simulink model "massignment2"  (Simulink 6.0)
settings: Solver=FixedStepDiscrete  StartTime=0.0  StopTime=10.0  RelTol=1e-3
settings Model: Creator=awarlock  LastModifiedBy=awarlock  ExtModeAutoUpdateStatusClock=off
settings OptimizationCC: InlineParams=on
settings DebuggingCC: MultiTaskDSMMsg=warning

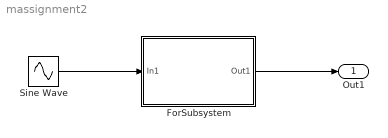
== system massignment2 ==
  ForSubsystem : Subsystem
  Sine Wave : Sin  Amplitude=3:7  SampleTime=0.1
  Out1 : Outport
  wires:
  Sine Wave/1 -> ForSubsystem/1(In1)
  ForSubsystem/1(Out1) -> Out1/1

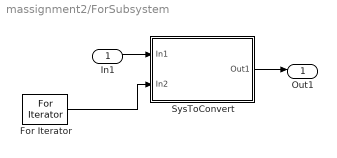
== system massignment2/ForSubsystem ==
  In1 : Inport  Port=1  LatchInput=off
  For Iterator : ForIterator  IterationVariableDataType=double
  SysToConvert : Subsystem  TreatAsAtomicUnit=on
  Out1 : Outport
  wires:
  In1/1 -> SysToConvert/1(In1)
  SysToConvert/1(Out1) -> Out1/1
  For Iterator/1 -> SysToConvert/2(In2)

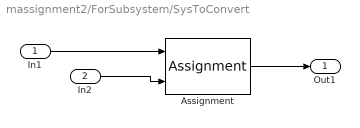
== system massignment2/ForSubsystem/SysToConvert ==
  In1 : Inport  Port=1  LatchInput=off
  In2 : Inport  Port=2  LatchInput=off
  Assignment : Assignment
  Out1 : Outport
  wires:
  In1/1 -> Assignment/1
  Assignment/1 -> Out1/1
  In2/1 -> Assignment/2
